simulink model "PID_FEScontrollerSim"  (R2020b)
settings: Solver=VariableStepAuto  StartTime=0.0  StopTime=100000  RelTol=1e-3
values from neighbouring files (symbols this model uses):
  h_mdls = calibration(elecArray, maxStimAmp, maxForce,h_mdl_struct, bt)    [FES_open_loop.m]
libraries: dspnetwork x4, slident x3, pid_lib x2, sldrtlib x1
settings Model: Creator=ayurkewi  LastModifiedBy=Wacom hrg
settings DataIOCC: ReturnWorkspaceOutputs=off
settings DebuggingCC: ArithmeticOperatorsInVariantConditions=warning
settings SFSimCC: CustomCodeUndefinedFunction=UseInterfaceOnly

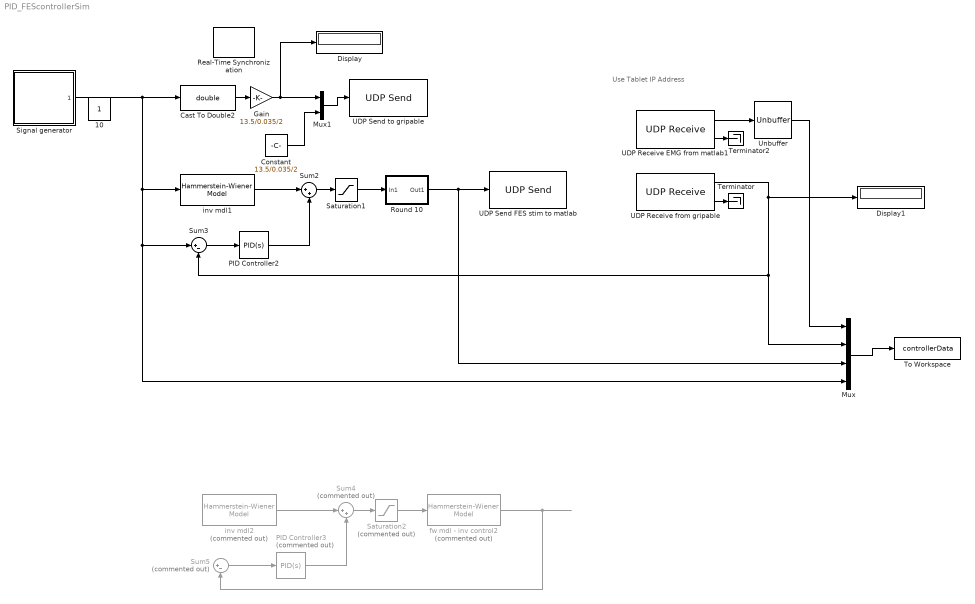
== system PID_FEScontrollerSim ==
  note: Use Tablet IP Address
  Cast To Double2 : DataTypeConversion  OutDataTypeStr=double
  Constant : Constant  Value=13.5/0.035/2
  Display : Display
  Display1 : Display
  Gain : Gain  Gain=13.5/0.035/2
  Mux : Mux
  Mux1 : Mux  Inputs=2
  PID Controller2 : pid_lib/PID Controller  Controller=PID  Form=Parallel  TimeDomain=Continuous-time  UseExternalTs=off  SampleTime=-1  IntegratorMethod=Forward Euler  FilterMethod=Forward Euler  ControllerParametersSource=internal  P=5000  I=0  D=0  UseFilter=on  N=1  TunerSelectOption=Transfer Function Based (PID Tuner App)  InitialConditionSource=internal  InitialConditionForIntegrator=0  InitialConditionForFilter=0  DifferentiatorICPrevScaledInput=0  ExternalReset=none  TrackingMode=off  Kt=1  LimitOutput=off  SatLimitsSource=internal  UpperSaturationLimit=inf  LowerSaturationLimit=-inf  LinearizeAsGain=on  AntiWindupMode=none  Kb=1  POutMin=[]  POutMax=[]  IOutMin=[]  IOutMax=[]  DOutMin=[]  DOutMax=[]  NOutMin=[]  NOutMax=[]  SumOutMin=[]  SumOutMax=[]  SaturationOutMin=[]  SaturationOutMax=[]  PParamMin=[]  PParamMax=[]  IParamMin=[]  IParamMax=[]  DParamMin=[]  DParamMax=[]  NParamMin=[]  NParamMax=[]  KbParamMin=[]  KbParamMax=[]  KtParamMin=[]  KtParamMax=[]  KbOutMin=[]  KbOutMax=[]  KtOutMin=[]  KtOutMax=[]  IntegratorOutMin=[]  IntegratorOutMax=[]  FilterOutMin=[]  FilterOutMax=[]  SumI1OutMin=[]  SumI1OutMax=[]  SumI2OutMin=[]  SumI2OutMax=[]  SumI3OutMin=[]  SumI3OutMax=[]  SumI4OutMin=[]  SumI4OutMax=[]  SumDOutMin=[]  SumDOutMax=[]  DifferentiatorOutMin=[]  DifferentiatorOutMax=[]  FilterDiffOutCoefMin=[]  FilterDiffOutCoefMax=[]  ReciprocalOutMin=[]  ReciprocalOutMax=[]  SumDenOutMin=[]  SumDenOutMax=[]  SumNumOutMin=[]  SumNumOutMax=[]  DivideOutMin=[]  DivideOutMax=[]  UdiffTsProdOutMin=[]  UdiffTsProdOutMax=[]  NTsProdOutMin=[]  NTsProdOutMax=[]  UintegralTsProdOutMin=[]  UintegralTsProdOutMax=[]  UngainTsProdOutMin=[]  UngainTsProdOutMax=[]  IntegratorContinuousStateAttributes=''  IntegratorStateMustResolveToSignalObject=off  IntegratorRTWStateStorageClass=Auto  FilterContinuousStateAttributes=''  FilterStateMustResolveToSignalObject=off  FilterRTWStateStorageClass=Auto  ParallelPVariant=InternalParameters  IdealPVariant=Disabled  IVariant=InternalParameters  DVariant=InternalParameters  IntegratorVariant=Continuous  SatVariant=Disabled  AWVariant=Passthrough  PCopyVariant=Disabled  TRVariant=Disabled  FdbkBlocksVariant=Forward  IdealPFdbkVariant=Disabled  SatFdbkVariant=Disabled  DerivativeFilterVariant=ContFilter  NVariant=InternalParameters  NCopyVariant=Disabled  FilterICVariant=InternalICsFilter  IntegratorICVariant=InternalICs  ExternalResetVariant=Disabled  TRSumVariant=Passthrough  SumFdbkVariant=Disabled  SumVariant=Sum_PID  TsampFilterVariant=InternalTs  TsampNgainVariant=Passthrough  TsampIntegralVariant=Passthrough  ExternalSaturationOutDataTypeStr=Inherit: Same as second input
  PID Controller3 : pid_lib/PID Controller  Commented=on  Controller=PID  Form=Parallel  TimeDomain=Continuous-time  UseExternalTs=off  SampleTime=-1  IntegratorMethod=Forward Euler  FilterMethod=Forward Euler  ControllerParametersSource=internal  P=-4436.19382448454  I=-12050.8903411551  D=50.4644378566483  UseFilter=on  N=5.1948030325436  TunerSelectOption=Transfer Function Based (PID Tuner App)  InitialConditionSource=internal  InitialConditionForIntegrator=0  InitialConditionForFilter=0  DifferentiatorICPrevScaledInput=0  ExternalReset=none  TrackingMode=off  Kt=1  LimitOutput=off  SatLimitsSource=internal  UpperSaturationLimit=inf  LowerSaturationLimit=-inf  LinearizeAsGain=on  AntiWindupMode=none  Kb=1  POutMin=[]  POutMax=[]  IOutMin=[]  IOutMax=[]  DOutMin=[]  DOutMax=[]  NOutMin=[]  NOutMax=[]  SumOutMin=[]  SumOutMax=[]  SaturationOutMin=[]  SaturationOutMax=[]  PParamMin=[]  PParamMax=[]  IParamMin=[]  IParamMax=[]  DParamMin=[]  DParamMax=[]  NParamMin=[]  NParamMax=[]  KbParamMin=[]  KbParamMax=[]  KtParamMin=[]  KtParamMax=[]  KbOutMin=[]  KbOutMax=[]  KtOutMin=[]  KtOutMax=[]  IntegratorOutMin=[]  IntegratorOutMax=[]  FilterOutMin=[]  FilterOutMax=[]  SumI1OutMin=[]  SumI1OutMax=[]  SumI2OutMin=[]  SumI2OutMax=[]  SumI3OutMin=[]  SumI3OutMax=[]  SumI4OutMin=[]  SumI4OutMax=[]  SumDOutMin=[]  SumDOutMax=[]  DifferentiatorOutMin=[]  DifferentiatorOutMax=[]  FilterDiffOutCoefMin=[]  FilterDiffOutCoefMax=[]  ReciprocalOutMin=[]  ReciprocalOutMax=[]  SumDenOutMin=[]  SumDenOutMax=[]  SumNumOutMin=[]  SumNumOutMax=[]  DivideOutMin=[]  DivideOutMax=[]  UdiffTsProdOutMin=[]  UdiffTsProdOutMax=[]  NTsProdOutMin=[]  NTsProdOutMax=[]  UintegralTsProdOutMin=[]  UintegralTsProdOutMax=[]  UngainTsProdOutMin=[]  UngainTsProdOutMax=[]  IntegratorContinuousStateAttributes=''  IntegratorStateMustResolveToSignalObject=off  IntegratorRTWStateStorageClass=Auto  FilterContinuousStateAttributes=''  FilterStateMustResolveToSignalObject=off  FilterRTWStateStorageClass=Auto  ParallelPVariant=InternalParameters  IdealPVariant=Disabled  IVariant=InternalParameters  DVariant=InternalParameters  IntegratorVariant=Continuous  SatVariant=Disabled  AWVariant=Passthrough  PCopyVariant=Disabled  TRVariant=Disabled  FdbkBlocksVariant=Forward  IdealPFdbkVariant=Disabled  SatFdbkVariant=Disabled  DerivativeFilterVariant=ContFilter  NVariant=InternalParameters  NCopyVariant=Disabled  FilterICVariant=InternalICsFilter  IntegratorICVariant=InternalICs  ExternalResetVariant=Disabled  TRSumVariant=Passthrough  SumFdbkVariant=Disabled  SumVariant=Sum_PID  TsampFilterVariant=InternalTs  TsampNgainVariant=Passthrough  TsampIntegralVariant=Passthrough  ExternalSaturationOutDataTypeStr=Inherit: Same as second input
  Real-Time Synchronization : sldrtlib/Real-Time Synchronization  SampleTime=0.001  MaxMissedTicks=100000  ShowMissedTicks=off  YieldWhenWaiting=off
  Round 10 : Subsystem
  Saturation1 : Saturate  UpperLimit=400  LowerLimit=100
  Saturation2 : Saturate  Commented=on  UpperLimit=400  LowerLimit=100
  "Signal generator " : Subsystem  ReferencedSubsystem=Signal_generator_hi5
  Sum2 : Sum  Inputs=|++
  Sum3 : Sum  Inputs=|+-
  Sum4 : Sum  Commented=on  Inputs=|++
  Sum5 : Sum  Commented=on  Inputs=|+-
  Terminator : Terminator
  Terminator2 : Terminator
  To Workspace : ToWorkspace  VariableName=controllerData  SaveFormat=Timeseries  SampleTime=0.1
  UDP Receive EMG from matlab1 : dspnetwork/UDP Receive  localURL='0.0.0.0'  localPort=6000  remoteURL='0.0.0.0'  remotePort=-1  recvBufferSize=8192  dims=20  signalDatatype=double  isComplex=off  isVarSize=off  showBlockingTime=off  blockingTime=0  sampletime=0.020  blockPlatform=[]
  UDP Receive from gripable : dspnetwork/UDP Receive  localURL='0.0.0.0'  localPort=26000  remoteURL='0.0.0.0'  remotePort=-1  recvBufferSize=1024  dims=1  signalDatatype=double  isComplex=off  isVarSize=off  showBlockingTime=off  blockingTime=0  sampletime=0.01  blockPlatform=[]
  UDP Send FES stim to matlab : dspnetwork/UDP Send  remoteURL='127.0.0.1'  remotePort=22392  localURL='0.0.0.0'  localPortSource=Automatically determine  localPort=-1  sendBufferSize=8190  sampletime=-1  blockPlatform=[]  separateLengthPort=0
  UDP Send to gripable : dspnetwork/UDP Send  remoteURL='146.169.203.190'  remotePort=25000  localURL='0.0.0.0'  localPortSource=Automatically determine  localPort=-1  sendBufferSize=1  sampletime=-1  blockPlatform=[]  separateLengthPort=0
  Unbuffer : Unbuffer
  fw mdl - inv control2 : slident/Models/Hammerstein-Wiener Model  Commented=on  sys=mdl  IC=Zero  X0i=0
      settings: SourceProductBaseCode=ID
  inv mdl1 : slident/Models/Hammerstein-Wiener Model  sys=h_mdls{1}  IC=Zero  X0i=0
      settings: SourceProductBaseCode=ID
  inv mdl2 : slident/Models/Hammerstein-Wiener Model  Commented=on  sys=mdl2  IC=Zero  X0i=0
      settings: SourceProductBaseCode=ID
  10 : Constant  IOType=siggen
  wires:
  Cast To Double2/1 -> Gain/1
  UDP Receive from gripable/2 -> Terminator/1
  UDP Receive from gripable/1 -> Display1/1, Mux/2, Sum3/2
  Mux/1 -> To Workspace/1
  UDP Receive EMG from matlab1/2 -> Terminator2/1
  UDP Receive EMG from matlab1/1 -> Unbuffer/1
  "Signal generator "/1 -> Mux/4, Sum3/1, inv mdl1/1, Cast To Double2/1
  Sum2/1 -> Saturation1/1
  inv mdl1/1 -> Sum2/1
  PID Controller2/1 -> Sum2/2
  Sum3/1 -> PID Controller2/1
  inv mdl2/1 -> Sum4/1
  Sum4/1 -> Saturation2/1
  PID Controller3/1 -> Sum4/2
  Sum5/1 -> PID Controller3/1
  Saturation2/1 -> fw mdl - inv control2/1
  fw mdl - inv control2/1 -> Sum5/2
  Unbuffer/1 -> Mux/1
  ? -> Sum5/1, inv mdl2/1
  Gain/1 -> Mux1/1, Display/1
  Mux1/1 -> UDP Send to gripable/1
  Constant/1 -> Mux1/2
  Round 10/1(Out1) -> UDP Send FES stim to matlab/1, Mux/3
  Saturation1/1 -> Round 10/1(In1)

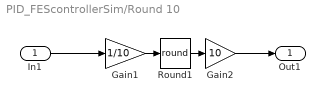
== system PID_FEScontrollerSim/Round 10 ==
  In1 : Inport
  Gain1 : Gain  Gain=1/10
  Gain2 : Gain  Gain=10
  Round1 : Rounding  Operator=round
  Out1 : Outport
  wires:
  Round1/1 -> Gain2/1
  Gain1/1 -> Round1/1
  In1/1 -> Gain1/1
  Gain2/1 -> Out1/1
